simulink model "untitled"  (R2016b)
settings: Solver=VariableStepAuto  StartTime=0.0  StopTime=100  RelTol=1e-3
values from neighbouring files (symbols this model uses):
  Ul = -1 : 0.01 : 1    [zad1_dod.m]    (also in zad6.m = -0.5)
undefined symbols (not defined in the file or in its folder): Tp
settings Model: Creator=tomasz  LastModifiedBy=tomasz

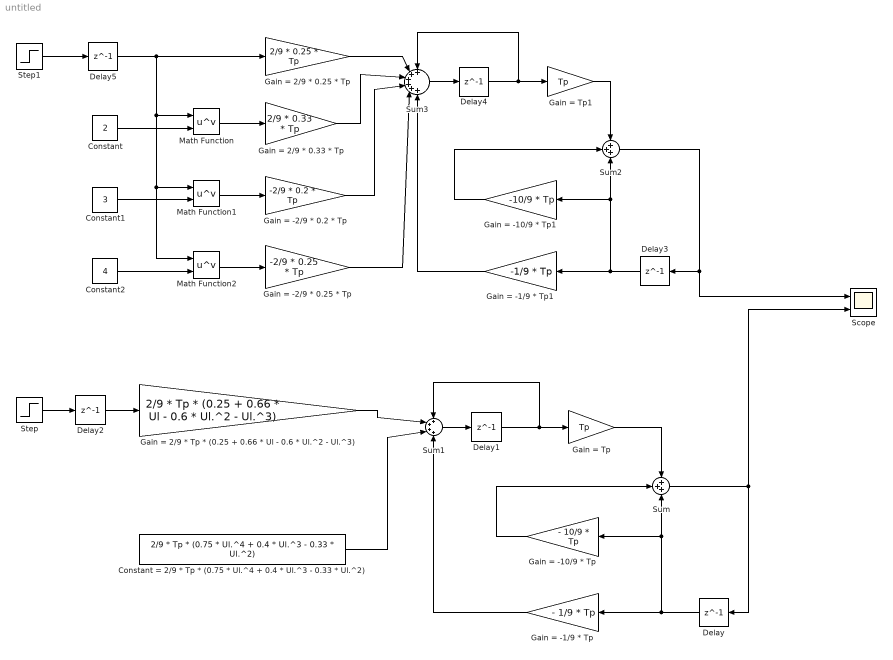
== system untitled ==
  Constant : Constant  Value=2
  Constant = 2/9 * Tp * (0.75 * Ul.^4 + 0.4 * Ul.^3 - 0.33 * Ul.^2) : Constant  Value=2/9 * Tp * (0.75 * Ul.^4 + 0.4 * Ul.^3 - 0.33 * Ul.^2)
  Constant1 : Constant  Value=3
  Constant2 : Constant  Value=4
  Delay{,1..5} (6 alike) : Delay  DelayLength=1  InitialCondition=0  SampleTime=Tp
  Gain = -1/9 * Tp : Gain  Gain=- 1/9 * Tp
  Gain = -1/9 * Tp1 : Gain  Gain=-1/9 * Tp
  Gain = -10/9 * Tp : Gain  Gain=- 10/9 * Tp
  Gain = -10/9 * Tp1 : Gain  Gain=-10/9 * Tp
  Gain = -2/9 * 0.2 * Tp : Gain  Gain=-2/9 * 0.2 * Tp
  Gain = -2/9 * 0.25 * Tp : Gain  Gain=-2/9 * 0.25 * Tp
  Gain = 2/9 * 0.25 * Tp : Gain  Gain=2/9 * 0.25 * Tp
  Gain = 2/9 * 0.33 * Tp : Gain  Gain=2/9 * 0.33 * Tp
  Gain = 2/9 * Tp * (0.25 + 0.66 * Ul - 0.6 * Ul.^2 - Ul.^3) : Gain  Gain=2/9 * Tp * (0.25 + 0.66 * Ul - 0.6 * Ul.^2 - Ul.^3)
  Gain = Tp : Gain  Gain=Tp
  Gain = Tp1 : Gain  Gain=Tp
  Math Function : Math  Operator=pow  SaturateOnIntegerOverflow=on
  Math Function1 : Math  Operator=pow  SaturateOnIntegerOverflow=on
  Math Function2 : Math  Operator=pow  SaturateOnIntegerOverflow=on
  Scope : Scope  NumInputPorts=2
  Step : Step  After=Ul  SampleTime=Tp
  Step1 : Step  After=Ul  SampleTime=Tp
  Sum : Sum  Inputs=+++
  Sum1 : Sum  Inputs=++++
  Sum2 : Sum  Inputs=+++
  Sum3 : Sum  Inputs=++++++
  wires:
  Sum/1 -> Scope/2, Delay/1
  Delay1/1 -> Sum1/1, Gain = Tp/1
  Delay/1 -> Gain = -1/9 * Tp/1, Gain = -10/9 * Tp/1, Sum/3
  Gain = -10/9 * Tp/1 -> Sum/2
  Gain = Tp/1 -> Sum/1
  Sum1/1 -> Delay1/1
  Gain = -1/9 * Tp/1 -> Sum1/4
  Step/1 -> Delay2/1
  Delay2/1 -> Gain = 2/9 * Tp * (0.25 + 0.66 * Ul - 0.6 * Ul.^2 - Ul.^3)/1
  Gain = 2/9 * Tp * (0.25 + 0.66 * Ul - 0.6 * Ul.^2 - Ul.^3)/1 -> Sum1/2
  Constant = 2/9 * Tp * (0.75 * Ul.^4 + 0.4 * Ul.^3 - 0.33 * Ul.^2)/1 -> Sum1/3
  Delay3/1 -> Sum2/3, Gain = -10/9 * Tp1/1, Gain = -1/9 * Tp1/1
  Sum2/1 -> Scope/1, Delay3/1
  Gain = -10/9 * Tp1/1 -> Sum2/2
  Sum3/1 -> Delay4/1
  Delay4/1 -> Sum3/1, Gain = Tp1/1
  Gain = Tp1/1 -> Sum2/1
  Gain = -1/9 * Tp1/1 -> Sum3/6
  Constant2/1 -> Math Function2/2
  Constant1/1 -> Math Function1/2
  Constant/1 -> Math Function/2
  Delay5/1 -> Math Function2/1, Math Function1/1, Math Function/1, Gain = 2/9 * 0.25 * Tp/1
  Gain = 2/9 * 0.25 * Tp/1 -> Sum3/2
  Math Function/1 -> Gain = 2/9 * 0.33 * Tp/1
  Gain = 2/9 * 0.33 * Tp/1 -> Sum3/3
  Math Function2/1 -> Gain = -2/9 * 0.25 * Tp/1
  Math Function1/1 -> Gain = -2/9 * 0.2 * Tp/1
  Gain = -2/9 * 0.2 * Tp/1 -> Sum3/4
  Gain = -2/9 * 0.25 * Tp/1 -> Sum3/5
  Step1/1 -> Delay5/1
